simulink model "BuildingModelWithSolarLoadAndHVAC"  (R2025a)
settings: Solver=daessc  StartTime=0.0  StopTime=604800  FixedStep=60*15  MaxStep=60  RelTol=1e-3  AbsTol=1e-3
PreLoadFcn:
  | % WallModelParams
libraries: nesl_utility x12, fl_lib x6, slpidlib x1
(part 2 of 2)

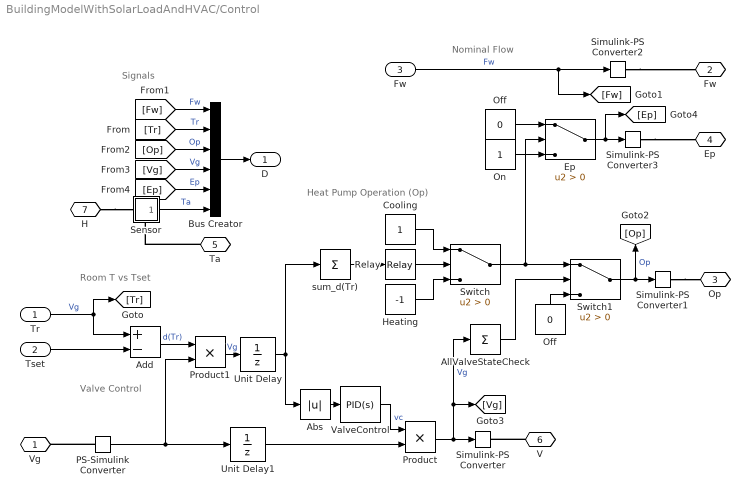
== system BuildingModelWithSolarLoadAndHVAC/Control ==
  note: Signals
  note: Nominal Flow
  note: Heat Pump Operation (Op)
  note: Room T vs Tset
  note: Valve Control
  Tr : Inport
  Tset : Inport  Port=2
  Fw : Inport  Port=3
  Abs : Abs  SaturateOnIntegerOverflow=off
  Add : Sum  Inputs=+-
  AllValveStateCheck : Sum  Inputs=+
  Bus Creator : BusCreator  Inputs=6
  Cooling : Constant
  Ep : Switch  Criteria=u2 > Threshold  SaturateOnIntegerOverflow=off  InputSameDT=off
  Heating : Constant  Value=-1
  Off : Constant  Value=0
  "Off " : Constant  Value=0
  On : Constant
  PS-Simulink Converter : nesl_utility/PS-Simulink Converter  PhysicalDomain=network_engine_domain  SubClassName=ps_output  LeftPortType=input  RightPortType=output  PseudoPeriodic=off  Frequencies=[]  VectorFormat=inherit  Unit=inherit  AffineConversion=off
  Product : Product
  Product1 : Product
  Relay : Relay  OnSwitchValue=1  OffSwitchValue=-1
  Sensor : Subsystem
      settings: PortSchema="{\"entries\":[{\"content\":{\"sides\":[{\"content\":{\"connectorIds\":[\"Out1\"]},\"type\":\"ConnectorPlacement.EquallySpacedRectSide\",\"uuid\":\"b4a62496-ee0e-470a-8e11-b80ed15f57a3\"},{\"content\":{\"connectorIds\":[\"RConn1\"],\"side\":\"RIGHT\"},\"type\":\"ConnectorPlacement.EquallySpacedRectSide\",\"uuid\":\"ca6e1c51-e9c2-402f-85b0-472d3ab7fde7\"},{\"content\":{\"connectorIds\":[\"LConn1\"],\"side\":\"TOP\"},\"type\":\"ConnectorPlacement.EquallySpacedRectSide\",\"uuid\":\"decc8abd-c589-4bdb-8a36-e72094d94d93\"},{\"content\":{\"side\":\"BOTTOM\"},\"type\":\"ConnectorPlacement.EquallySpacedRectSide\",\"uuid\":\"9abf708e-9771-4262-8a2d-bc8c207678cd\"}]},\"type\":\"ConnectorPlacement.EquallySpacedConnector\",\"uuid\":\"a0fe939d-cd8d-45fe-af96-db4e47edfd06\"}],\"packageUris\":[\"http://schema.mathworks.com/mf0/Connector/R2020b\"],\"version\":\"1.0\"}"
  Simulink-PS Converter : nesl_utility/Simulink-PS Converter  PhysicalDomain=network_engine_domain  SubClassName=ps_input  LeftPortType=input  RightPortType=output  PseudoPeriodic=off  Frequencies=[]  NoiseDistribution=none  NoiseParameters=[]  Unit=1  AffineConversion=off  FilteringAndDerivatives=filter  SimscapeFilterOrder=1  InputFilterTimeConstant=0.001  UdotUserProvided=0
  Simulink-PS Converter1 : nesl_utility/Simulink-PS Converter  PhysicalDomain=network_engine_domain  SubClassName=ps_input  LeftPortType=input  RightPortType=output  PseudoPeriodic=off  Frequencies=[]  NoiseDistribution=none  NoiseParameters=[]  Unit=1  AffineConversion=off  FilteringAndDerivatives=filter  SimscapeFilterOrder=1  InputFilterTimeConstant=0.001  UdotUserProvided=0
  Simulink-PS Converter2 : nesl_utility/Simulink-PS Converter  PhysicalDomain=network_engine_domain  SubClassName=ps_input  LeftPortType=input  RightPortType=output  PseudoPeriodic=off  Frequencies=[]  NoiseDistribution=none  NoiseParameters=[]  Unit=kg/s  AffineConversion=off  FilteringAndDerivatives=filter  SimscapeFilterOrder=1  InputFilterTimeConstant=0.001  UdotUserProvided=0
  Simulink-PS Converter3 : nesl_utility/Simulink-PS Converter  PhysicalDomain=network_engine_domain  SubClassName=ps_input  LeftPortType=input  RightPortType=output  PseudoPeriodic=off  Frequencies=[]  NoiseDistribution=none  NoiseParameters=[]  Unit=1  AffineConversion=off  FilteringAndDerivatives=filter  SimscapeFilterOrder=1  InputFilterTimeConstant=0.001  UdotUserProvided=0
  Switch : Switch  Criteria=u2 > Threshold  SaturateOnIntegerOverflow=off  InputSameDT=off
  Switch1 : Switch  Criteria=u2 > Threshold  SaturateOnIntegerOverflow=off  InputSameDT=off
  Unit Delay : UnitDelay  SampleTime=-1  HasFrameUpgradeWarning=on
  Unit Delay1 : UnitDelay  InitialCondition=1  SampleTime=-1  HasFrameUpgradeWarning=on
  ValveControl : slpidlib/PID Controller  Controller=PID  Form=Parallel  TimeDomain=Continuous-time  UseExternalTs=off  SampleTime=-1  IntegratorMethod=Forward Euler  FilterMethod=Forward Euler  ControllerParametersSource=internal  P=0.5  I=0.1  UseKiTs=off  D=0  UseExternalDerivativeSource=off  N=0  UseFilter=on  TunerSelectOption=Transfer Function Based (PID Tuner App)  InitialConditionSource=internal  InitialConditionForIntegrator=0.1  InitialConditionForFilter=0.1  DifferentiatorICPrevScaledInput=0  ExternalReset=none  TrackingMode=off  Kt=1  LimitOutput=on  SatLimitsSource=internal  UpperSaturationLimit=1  LowerSaturationLimit=0  LinearizeAsGain=on  AntiWindupMode=none  Kb=1  LimitIntegrator=on  UpperIntegratorSaturationLimit=1.1  LowerIntegratorSaturationLimit=0.1  POutMin=[]  POutMax=[]  IOutMin=[]  IOutMax=[]  DOutMin=[]  DOutMax=[]  NOutMin=[]  NOutMax=[]  SumOutMin=[]  SumOutMax=[]  SaturationOutMin=[]  SaturationOutMax=[]  PParamMin=[]  PParamMax=[]  IParamMin=[]  IParamMax=[]  DParamMin=[]  DParamMax=[]  NParamMin=[]  NParamMax=[]  KbParamMin=[]  KbParamMax=[]  KtParamMin=[]  KtParamMax=[]  KbOutMin=[]  KbOutMax=[]  KtOutMin=[]  KtOutMax=[]  IntegratorOutMin=[]  IntegratorOutMax=[]  FilterOutMin=[]  FilterOutMax=[]  SumI1OutMin=[]  SumI1OutMax=[]  SumI2OutMin=[]  SumI2OutMax=[]  SumI3OutMin=[]  SumI3OutMax=[]  SumI4OutMin=[]  SumI4OutMax=[]  SumDOutMin=[]  SumDOutMax=[]  DifferentiatorOutMin=[]  DifferentiatorOutMax=[]  FilterDiffOutCoefMin=[]  FilterDiffOutCoefMax=[]  ReciprocalOutMin=[]  ReciprocalOutMax=[]  SumDenOutMin=[]  SumDenOutMax=[]  SumNumOutMin=[]  SumNumOutMax=[]  DivideOutMin=[]  DivideOutMax=[]  UdiffTsProdOutMin=[]  UdiffTsProdOutMax=[]  NTsProdOutMin=[]  NTsProdOutMax=[]  UintegralTsProdOutMin=[]  UintegralTsProdOutMax=[]  UngainTsProdOutMin=[]  UngainTsProdOutMax=[]  ClampingZeroOutDataTypeStr=Inherit: Inherit via back propagation  ClampingZeroOutMin=[]  ClampingZeroOutMax=[]  FilterDenConstantOutDataTypeStr=Inherit: Inherit via back propagation  FilterDenConstantOutMin=[]  FilterDenConstantOutMax=[]  PCopyOutDataTypeStr=Inherit: Inherit via back propagation  PCopyOutMin=[]  PCopyOutMax=[]  NCopyOutDataTypeStr=Inherit: Inherit via back propagation  NCopyOutMin=[]  NCopyOutMax=[]  IntegratorContinuousStateAttributes=''  IntegratorStateMustResolveToSignalObject=off  IntegratorRTWStateStorageClass=Auto  FilterContinuousStateAttributes=''  FilterStateMustResolveToSignalObject=off  FilterRTWStateStorageClass=Auto  ParallelPVariant=InternalParameters  IdealPVariant=Disabled  IVariant=InternalParameters  DVariant=InternalParameters  IntegratorVariant=Continuous  SatVariant=Enabled  AWVariant=Passthrough  PCopyVariant=Disabled  TRVariant=Disabled  FdbkBlocksVariant=Forward  IdealPFdbkVariant=Disabled  SatFdbkVariant=Disabled  DerivativeFilterVariant=ContFilter  NVariant=InternalParameters  NCopyVariant=Disabled  FilterICVariant=InternalICsFilter  IntegratorICVariant=InternalICs  ExternalResetVariant=Disabled  TRSumVariant=Passthrough  SumFdbkVariant=Disabled  SumVariant=Sum_PID  TsampFilterVariant=InternalTs  TsampNgainVariant=Passthrough  TsampIntegralVariant=Disabled_SignalSpec  ExternalSaturationOutDataTypeStr=Inherit: Same as second input  DerivativeSourceVariant=ErrorSignal  PreIntVariant=InternalPreInt
  sum_d(Tr) : Sum  Inputs=+
  Vg : PMIOPort  Side=Left
  "Fw " : PMIOPort  Port=2  Side=Left
  "Op " : PMIOPort  Port=3  Side=Left
  "Ep " : PMIOPort  Port=4  Side=Left
  Ta : PMIOPort  Port=5  Side=Left
  V : PMIOPort  Port=6  Side=Right
  H : PMIOPort  Port=7  Side=Right
  D : Outport
  wires:
  Tset/1 -> Add/2
  Bus Creator/1 -> D/1
  Product/1 -> Simulink-PS Converter/1, AllValveStateCheck/1, [Vg]  "Vg"
  sum_d(Tr)/1 -> Relay/1
  Cooling/1 -> Switch/1
  Heating/1 -> Switch/3
  Off/1 -> Switch1/3
  PS-Simulink Converter/1 -> Product1/2, Unit Delay1/1
  ValveControl/1 -> Product/1  "vc"
  Switch1/1 -> Simulink-PS Converter1/1, [Op]  "Op"
  [Tr] -> Bus Creator/2  "Tr"
  [Fw] -> Bus Creator/1  "Fw"
  [Op] -> Bus Creator/3  "Op"
  [Vg] -> Bus Creator/4  "Vg"
  Switch/1 -> Ep/2, Switch1/1
  Relay/1 -> Switch/2
  AllValveStateCheck/1 -> Switch1/2
  Fw/1 -> [Fw], Simulink-PS Converter2/1  "Fw"
  Tr/1 -> Add/1, [Tr]  "Vg"
  Unit Delay/1 -> sum_d(Tr)/1, Abs/1
  Unit Delay1/1 -> Product/2
  Abs/1 -> ValveControl/1
  "Off "/1 -> Ep/1
  On/1 -> Ep/3
  Ep/1 -> [Ep], Simulink-PS Converter3/1
  Sensor/1("  ") -> Bus Creator/6  "Ta"
  [Ep] -> Bus Creator/5  "Ep"
  Add/1 -> Product1/1  "d(Tr)"
  Product1/1 -> Unit Delay/1  "Vg"
  connections:
  V/RConn1 -- Simulink-PS Converter/RConn1
  Simulink-PS Converter1/RConn1 -- "Op "/RConn1
  Simulink-PS Converter2/RConn1 -- "Fw "/RConn1
  Simulink-PS Converter3/RConn1 -- "Ep "/RConn1
  H/RConn1 -- Sensor/RConn1
  Ta/RConn1 -- Sensor/LConn1
  PS-Simulink Converter/LConn1 -- Vg/RConn1

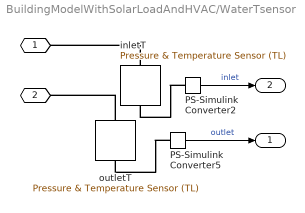
== system BuildingModelWithSolarLoadAndHVAC/WaterTsensor ==
  PS-Simulink Converter2 : nesl_utility/PS-Simulink Converter  PhysicalDomain=network_engine_domain  SubClassName=ps_output  LeftPortType=input  RightPortType=output  PseudoPeriodic=off  Frequencies=[]  VectorFormat=inherit  Unit=inherit  AffineConversion=off
  PS-Simulink Converter5 : nesl_utility/PS-Simulink Converter  PhysicalDomain=network_engine_domain  SubClassName=ps_output  LeftPortType=input  RightPortType=output  PseudoPeriodic=off  Frequencies=[]  VectorFormat=inherit  Unit=inherit  AffineConversion=off
  inletT : fl_lib/Thermal Liquid/Sensors/Pressure & Temperature Sensor (TL)  reference=foundation.enum.MeasurementReference.absolute  pressure=false  pressure_spec=foundation.enum.PressureMeasementSpec.Absolute  temperature=true
      settings: InternalSimscapePortConfiguration="{\"Bottom\":[{\"id\":\"T\",\"label\":\"T\",\"type\":\"output\"}],\"Left\":[{\"id\":\"A\",\"label\":\"A\",\"type\":\"foundation.thermal_liquid.thermal_liquid\"}],\"Right\":[],\"Top\":[]}"
  outletT : fl_lib/Thermal Liquid/Sensors/Pressure & Temperature Sensor (TL)  reference=foundation.enum.MeasurementReference.absolute  pressure=false  pressure_spec=foundation.enum.PressureMeasementSpec.Absolute  temperature=true
      settings: InternalSimscapePortConfiguration="{\"Bottom\":[{\"id\":\"T\",\"label\":\"T\",\"type\":\"output\"}],\"Left\":[{\"id\":\"A\",\"label\":\"A\",\"type\":\"foundation.thermal_liquid.thermal_liquid\"}],\"Right\":[],\"Top\":[]}"
  "  " : PMIOPort  Side=Left
  " " : PMIOPort  Port=2  Side=Left
  "    " : Outport
  "   " : Outport  Port=2
  wires:
  PS-Simulink Converter2/1 -> "   "/1  "inlet"
  PS-Simulink Converter5/1 -> "    "/1  "outlet"
  connections:
  PS-Simulink Converter2/LConn1 -- inletT/RConn1
  PS-Simulink Converter5/LConn1 -- outletT/RConn1
  inletT/LConn1 -- "  "/RConn1
  outletT/LConn1 -- " "/RConn1

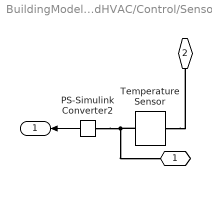
== system BuildingModelWithSolarLoadAndHVAC/Control/Sensor ==
  PS-Simulink Converter2 : nesl_utility/PS-Simulink Converter  PhysicalDomain=network_engine_domain  SubClassName=ps_output  LeftPortType=input  RightPortType=output  PseudoPeriodic=off  Frequencies=[]  VectorFormat=inherit  Unit=inherit  AffineConversion=off
  Temperature Sensor : fl_lib/Thermal/Thermal Sensors/Temperature Sensor  temperature_measure=foundation.enum.MeasurementReference.absolute
      settings: InternalSimscapePortConfiguration="{\"Bottom\":[],\"Left\":[{\"id\":\"A\",\"label\":\"A\",\"type\":\"foundation.thermal.thermal\"}],\"Right\":[{\"id\":\"T\",\"label\":\"T\",\"type\":\"output\"}],\"Top\":[]}"
  "   " : PMIOPort  Side=Left
  " " : PMIOPort  Port=2  Side=Right
  "  " : Outport
  wires:
  PS-Simulink Converter2/1 -> "  "/1
  connections:
  Temperature Sensor/LConn1 -- " "/RConn1
  Temperature Sensor/RConn1 -- "   "/RConn1 -- PS-Simulink Converter2/LConn1
